simulink model "model_main"  (R2023b)
settings: Solver=ode4  StartTime=0.0  StopTime=600  FixedStep=0.001  RelTol=1e-3
values from neighbouring files (symbols this model uses):
  RCS_THR_vec = [RCS1_THR,RCS2_THR,RCS3_THR,RCS4_THR,                          RCS5_THR,RCS6_THR,RCS7_THR,RCS8_THR,                          RCS9_THR,RCS10_THR,RCS11_THR,RCS12_THR]    [model_init.m]
  w_orbit = kepler6_to_orbit_rate(SC_Kepler)    [model_init.m]
undefined symbols (not defined in the file or in its folder): Fly_Wheel_Mass, RW_As, X, Y, Z
libraries: sm_lib x69, nesl_utility x48, simulink_extras x7, aerolibutil x4, sharedtransform x4
(part 2 of 2)

== matlab function model_main/MATLAB Function1 ==
  data: p_ref input; out output; p input; v_ref input; v input; RCS_THR_vec input
function out = fcn(p_ref, p, v_ref, v, RCS_THR_vec)
% ====== 파라미터 ======
Tmax   = 22;       % [N]
m = 2000;
% pwmMax = 65535;    % 예: 16-bit
% pwmMin = 0;        % 필요하면 최소 구동값 넣기
Kp = 20*diag([1 1 1]);
Kd = 40*diag([1 1 1]);
% ====== 1) PD -> F_cmd ======
e_p = p_ref - p;
e_v = v_ref - v;

a_cmd = Kp*e_p + Kd*e_v;
F_cmd = m * a_cmd;

% ====== 2) Allocation ======
% [u, F_ach] = rcs_allocate_lsqlin(F_cmd, RCS_THR_vec, Tmax); % toolbox 권장
[u, F_ach] = rcs_allocate_pinv_clip(F_cmd, RCS_THR_vec, Tmax); % 간단 대안

% ====== 3) PWM ======
% pwm = thrust_to_pwm(u, Tmax, pwmMax, pwmMin);
out = u./1;
% (디버그)
% disp("F_cmd  = " + mat2str(F_cmd',4))
% disp("F_ach  = " + mat2str(F_ach',4))
% disp("u(N)   = " + mat2str(u',4))
% disp("pwm    = " + mat2str(pwm',4))

end

function [u, F_ach] = rcs_allocate_pinv_clip(F_cmd, RCS_THR_vec, Tmax)
    B = RCS_THR_vec;     % 3xN
    u = pinv(B) * F_cmd; % unconstrained

    % Thruster는 보통 단방향(0~Tmax)이므로 음수는 0으로
    u = max(u, 0);
    u = min(u, Tmax);

    F_ach = B*u;
end


function pwm = thrust_to_pwm(u, Tmax, pwmMax, pwmMin)
    % u: Nx1 thrust command [N]
    % pwmMax: 예) 65535 또는 255
    % pwmMin: (선택) 밸브/드라이버가 실제로 열리는 최소 duty가 있으면 반영

    duty = u(:) / Tmax;          % 0~1
    duty = max(0, min(1, duty));

    if nargin >= 4 && pwmMin > 0
        % duty>0인 경우에만 최소 구동 듀티 적용(데드존)
        duty(duty>0) = max(duty(duty>0), pwmMin/pwmMax);
    end

    pwm = round(duty * pwmMax);
end

== matlab function model_main/MATLAB Function ==
  data: qe input; torq output; we input
function torq = fcn(qe, we)

K1 = 20.0 * diag([1 1 1]);
K2 = 800.0 * diag([1 1 1]);

qe_v = [qe(2), qe(3), qe(4)]';

torq = K1*qe_v + K2*we;

end

== matlab function model_main/MATLAB Function2 ==
  data: qe input; we input; As input; Omegad output
function Omegad = fcn(qe, we, As)

K1 = 5 * diag([1 1 1]);
K2 = 20.0 * diag([1 1 1]);

qe_v = [qe(2), qe(3), qe(4)]';

u = K1*qe_v + K2*we;

Iws = diag([0.00708857,0.00708857,0.00708857,0.00708857]);


Omegad = pinv(As*Iws)*-u;


end
